simulink model "pi_detect_circlered_hsv_onlyblock"  (R2016b)
settings: Solver=FixedStepAuto  StartTime=0.0  StopTime=1  RelTol=1e-3
undefined symbols (not defined in the file or in its folder): Rec, SDTV
libraries: visionconversions x5, embdlinuxlib x2, visiontextngfix x1
settings Model: SimulationMode=external  Creator=sk  LastModifiedBy=supak
settings SolverCC: PositivePriorityOrder=on
settings OptimizationCC: MaxStackSize=64
settings DebuggingCC: ParameterTunabilityLossMsg=error
settings HardwareCC: ProdBitPerPointer=32  ProdBitPerSizeT=32  ProdBitPerPtrDiffT=32  ProdLargestAtomicInteger=Long  ProdLargestAtomicFloat=Double  ProdWordSize=32  ProdHWDeviceType=ARM Compatible->ARM Cortex
settings RTWCC: SystemTargetFile=ert.tlc  HardwareBoard=Raspberry Pi  TLCOptions="-aInlineSetEventsForThisBaseRateFcn=TLC_FALSE -aSuppressMultiTaskScheduler=TLC_FALSE  -aRateBasedStepFcn=0"  TemplateMakefile=ert_default_tmf  Description=Embedded Coder  GenerateReport=on  Toolchain=GNU GCC Raspberry Pi  IncludeHyperlinkInReport=on  LaunchReport=on  GenerateTraceInfo=on  GenerateTraceReport=on  GenerateTraceReportSl=on  GenerateTraceReportSf=on  GenerateTraceReportEml=on
settings CodeAppCC: ForceParamTrailComments=on  IgnoreCustomStorageClasses=off  OperatorAnnotations=on  SimulinkDataObjDesc=on  SFDataObjDesc=on  MATLABFcnDesc=on  InsertBlockDesc=on  MATLABSourceComments=on
settings ERTTargetCC: SupportVariableSizeSignals=on

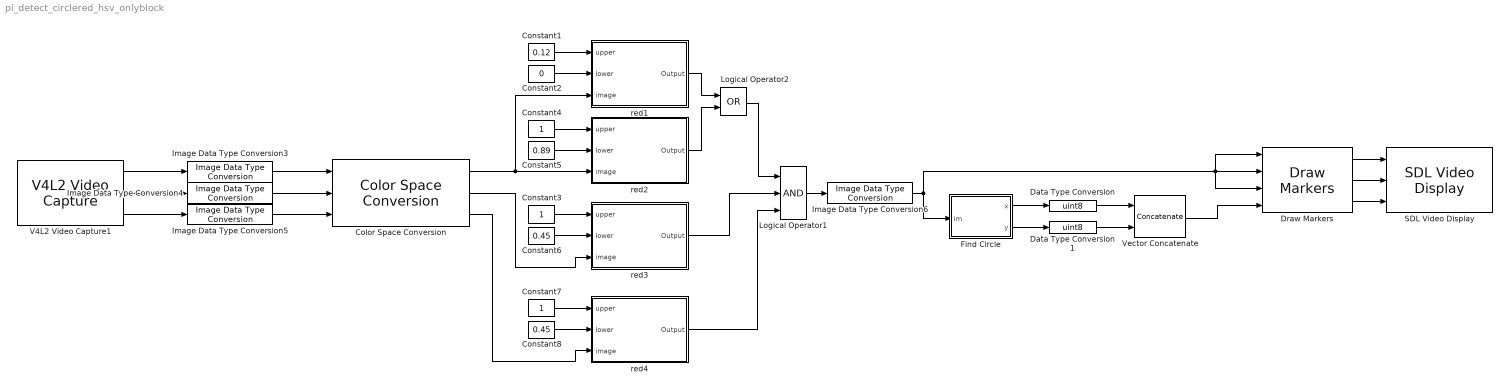
== system pi_detect_circlered_hsv_onlyblock ==
  Color Space Conversion : visionconversions/Color Space  Conversion  conversion=Obsolete  conversionActive=R'G'B' to HSV  wp_str=D65  rec=Rec. 601 (SDTV)  sys=1125/60/2:1  imagePorts=Separate color signals
  Constant1 : Constant  Value=0.12
  Constant2 : Constant  Value=0
  Constant3 : Constant
  Constant4 : Constant
  Constant5 : Constant  Value=0.89
  Constant6 : Constant  Value=0.45
  Constant7 : Constant
  Constant8 : Constant  Value=0.45
  Data Type Conversion : DataTypeConversion  OutDataTypeStr=uint8
  Data Type Conversion1 : DataTypeConversion  OutDataTypeStr=uint8
  Draw Markers : visiontextngfix/Draw Markers  shape=X-mark  size=5  fill=off  fillClrSource=Specify via dialog  display=Black  intensity=200  color=[200 255 100]  opacity=0.6  viewport=Entire image  antialiasing=off  inType=Obsolete  imagePorts=Separate color signals  prodOutputMode=Binary point scaling  prodOutputWordLength=32  prodOutputFracLength=14  memoryMode=Specify word length  memoryWordLength=16  memoryFracLength=15  roundingMode=Floor  overflowMode=off
  Find Circle : MATLAB Function  TreatAsAtomicUnit=on
  Image Data Type Conversion3 : visionconversions/Image Data Type Conversion  outDT=single  isSigned=on  wordLen=16  numFracBits=0
  Image Data Type Conversion4 : visionconversions/Image Data Type Conversion  outDT=single  isSigned=on  wordLen=16  numFracBits=0
  Image Data Type Conversion5 : visionconversions/Image Data Type Conversion  outDT=single  isSigned=on  wordLen=16  numFracBits=0
  Image Data Type Conversion6 : visionconversions/Image Data Type Conversion  outDT=uint8  isSigned=on  wordLen=16  numFracBits=0
  Logical Operator1 : Logic  Inputs=3  AllPortsSameDT=off  OutDataTypeStr=boolean
  Logical Operator2 : Logic  Operator=OR  AllPortsSameDT=off  OutDataTypeStr=boolean
  SDL Video Display : embdlinuxlib/SDL Video Display  pixelFormat=RGB  pixelOrder=Planar  rowMajor=on  blockPlatform=Raspberry Pi
  V4L2 Video Capture1 : embdlinuxlib/V4L2 Video Capture  m_devName='/dev/video0'  roi=[0, 0, 640, 480]  imSizeSelection=320x240  imSize=[640, 480]  pixelFormat=RGB  pixelOrder=Planar  sampleTime=1/10  simOutput=Colorbars  blockPlatform=Raspberry Pi
  Vector Concatenate : Concatenate  Mode=Multidimensional array
  red1 : Subsystem
  red2 : Subsystem
  red3 : Subsystem
  red4 : Subsystem
  wires:
  Image Data Type Conversion3/1 -> Color Space Conversion/1
  Image Data Type Conversion4/1 -> Color Space Conversion/2
  Image Data Type Conversion5/1 -> Color Space Conversion/3
  Logical Operator1/1 -> Image Data Type Conversion6/1
  V4L2 Video Capture1/1 -> Image Data Type Conversion3/1
  V4L2 Video Capture1/2 -> Image Data Type Conversion4/1
  V4L2 Video Capture1/3 -> Image Data Type Conversion5/1
  Image Data Type Conversion6/1 -> Draw Markers/3, Draw Markers/2, Draw Markers/1, Find Circle/1(im)
  Color Space Conversion/1 -> red1/3(image), red2/3(image)
  Constant1/1 -> red1/1(upper)
  Constant2/1 -> red1/2(Iower)
  Constant4/1 -> red2/1(upper)
  Constant5/1 -> red2/2(Iower)
  Color Space Conversion/2 -> red3/3(image)
  Constant3/1 -> red3/1(upper)
  Constant6/1 -> red3/2(Iower)
  Color Space Conversion/3 -> red4/3(image)
  Constant7/1 -> red4/1(upper)
  Constant8/1 -> red4/2(Iower)
  red1/1(Output) -> Logical Operator2/1
  red2/1(Output) -> Logical Operator2/2
  Logical Operator2/1 -> Logical Operator1/1
  red3/1(Output) -> Logical Operator1/2
  red4/1(Output) -> Logical Operator1/3
  Draw Markers/1 -> SDL Video Display/1
  Draw Markers/2 -> SDL Video Display/2
  Draw Markers/3 -> SDL Video Display/3
  Find Circle/1(x) -> Data Type Conversion/1
  Find Circle/2(y) -> Data Type Conversion1/1
  Vector Concatenate/1 -> Draw Markers/4
  Data Type Conversion/1 -> Vector Concatenate/1
  Data Type Conversion1/1 -> Vector Concatenate/2

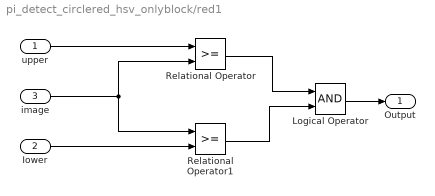
== system pi_detect_circlered_hsv_onlyblock/red1 ==
  upper : Inport
  Iower : Inport  Port=2
  image : Inport  Port=3
  Logical Operator : Logic  AllPortsSameDT=off  OutDataTypeStr=boolean
  Relational Operator : RelationalOperator  OutDataTypeStr=boolean  RndMeth=Simplest
  Relational Operator1 : RelationalOperator  OutDataTypeStr=boolean  RndMeth=Simplest
  Output : Outport
  wires:
  upper/1 -> Relational Operator/1
  Iower/1 -> Relational Operator1/2
  image/1 -> Relational Operator/2, Relational Operator1/1
  Relational Operator/1 -> Logical Operator/1
  Relational Operator1/1 -> Logical Operator/2
  Logical Operator/1 -> Output/1

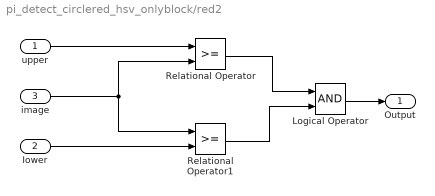
== system pi_detect_circlered_hsv_onlyblock/red2 ==
  upper : Inport
  Iower : Inport  Port=2
  image : Inport  Port=3
  Logical Operator : Logic  AllPortsSameDT=off  OutDataTypeStr=boolean
  Relational Operator : RelationalOperator  OutDataTypeStr=boolean  RndMeth=Simplest
  Relational Operator1 : RelationalOperator  OutDataTypeStr=boolean  RndMeth=Simplest
  Output : Outport
  wires:
  upper/1 -> Relational Operator/1
  Iower/1 -> Relational Operator1/2
  image/1 -> Relational Operator/2, Relational Operator1/1
  Relational Operator/1 -> Logical Operator/1
  Relational Operator1/1 -> Logical Operator/2
  Logical Operator/1 -> Output/1

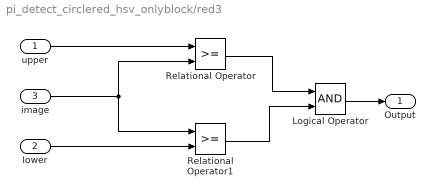
== system pi_detect_circlered_hsv_onlyblock/red3 ==
  upper : Inport
  Iower : Inport  Port=2
  image : Inport  Port=3
  Logical Operator : Logic  AllPortsSameDT=off  OutDataTypeStr=boolean
  Relational Operator : RelationalOperator  OutDataTypeStr=boolean  RndMeth=Simplest
  Relational Operator1 : RelationalOperator  OutDataTypeStr=boolean  RndMeth=Simplest
  Output : Outport
  wires:
  upper/1 -> Relational Operator/1
  Iower/1 -> Relational Operator1/2
  image/1 -> Relational Operator/2, Relational Operator1/1
  Relational Operator/1 -> Logical Operator/1
  Relational Operator1/1 -> Logical Operator/2
  Logical Operator/1 -> Output/1

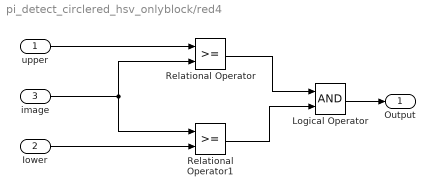
== system pi_detect_circlered_hsv_onlyblock/red4 ==
  upper : Inport
  Iower : Inport  Port=2
  image : Inport  Port=3
  Logical Operator : Logic  AllPortsSameDT=off  OutDataTypeStr=boolean
  Relational Operator : RelationalOperator  OutDataTypeStr=boolean  RndMeth=Simplest
  Relational Operator1 : RelationalOperator  OutDataTypeStr=boolean  RndMeth=Simplest
  Output : Outport
  wires:
  upper/1 -> Relational Operator/1
  Iower/1 -> Relational Operator1/2
  image/1 -> Relational Operator/2, Relational Operator1/1
  Relational Operator/1 -> Logical Operator/1
  Relational Operator1/1 -> Logical Operator/2
  Logical Operator/1 -> Output/1

== matlab function pi_detect_circlered_hsv_onlyblock/Find Circle ==
  data: im input; x output; y output
% Author : Supakit Kriangkhajorn
% Follow me : skconan
function [x,y]= findcircle(im)
    coder.extrinsic('imfindcircles'); 
    coder.extrinsic('isempty');
    coder.extrinsic('sortrows');
    coder.extrinsic('size');
    img = im;
    x = 150;
    y = 150;
    centerMax = [0,0];
    cols = 0;
%     radiusMax = 0;
    [centers, radius, metric] = imfindcircles(img,[35 65],'ObjectPolarity','bright');
    circles = [centers, radius, metric];
    check = ~isempty(circles)
    if check
        circles = sortrows(circles,3);
        [rows,cols] = size(circles);
        centerMax = circles(rows,1:2);
%         radiusMax = circles(rows,3);
    end
         
x = round(centerMax(1));
y = round(centerMax(2));
